simulink model "Alcantara_V_MATLAB_No1"  (R2023b)
settings: Solver=VariableStepAuto  StartTime=0.0  StopTime=10.0  RelTol=1e-3
settings Model: Creator=Vincent L. Alcantara  LastModifiedBy=Vincent L. Alcantara

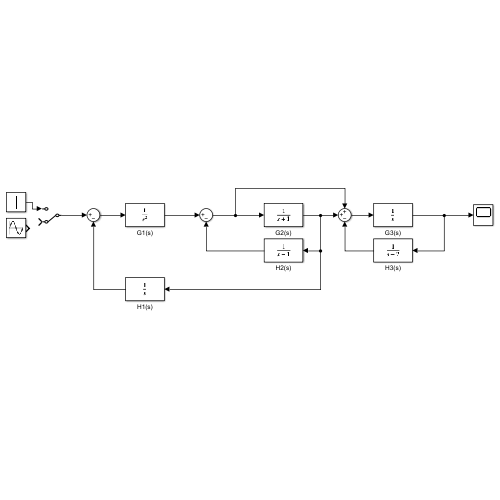
[thumbnail: Simulink's stored preview of the top-level diagram]
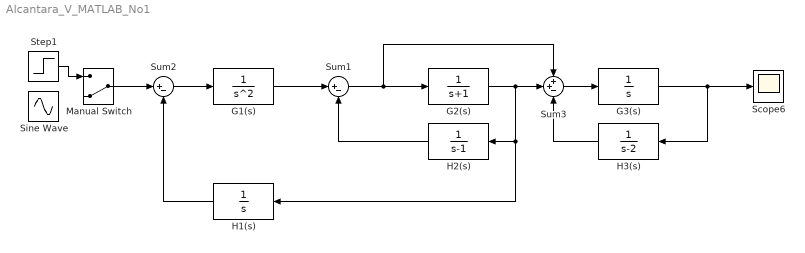
== system Alcantara_V_MATLAB_No1 ==
  G1(s) : TransferFcn  Denominator=[1 0 0]
  G2(s) : TransferFcn  Denominator=[1 1]
  G3(s) : TransferFcn  Denominator=[1 0]
  H1(s) : TransferFcn  Denominator=[1 0]
  H2(s) : TransferFcn  Denominator=[1 -1]
  H3(s) : TransferFcn  Denominator=[1 -2]
  Manual Switch : ManualSwitch  CurrentSetting=0
  Scope6 : Scope
  Sine Wave : Sin  SampleTime=0
  Step1 : Step  Time=0  SampleTime=0
  Sum1 : Sum  Inputs=|+-
  Sum2 : Sum  Inputs=|+-
  Sum3 : Sum  Inputs=++-
  wires:
  Manual Switch/1 -> Sum2/1
  G3(s)/1 -> H3(s)/1, Scope6/1
  H3(s)/1 -> Sum3/3
  Step1/1 -> Manual Switch/1
  Sum3/1 -> G3(s)/1
  H1(s)/1 -> Sum2/2
  G2(s)/1 -> H1(s)/1, H2(s)/1, Sum3/2
  H2(s)/1 -> Sum1/2
  Sum2/1 -> G1(s)/1
  Sum1/1 -> Sum3/1, G2(s)/1
  G1(s)/1 -> Sum1/1
